simulink model "simple_model"  (R2024a)
settings: Solver=VariableStepAuto  StartTime=0.0  StopTime=150  RelTol=1e-3
InitFcn:
  | A = 100 ;
settings Model: Creator=pc  LastModifiedBy=pc

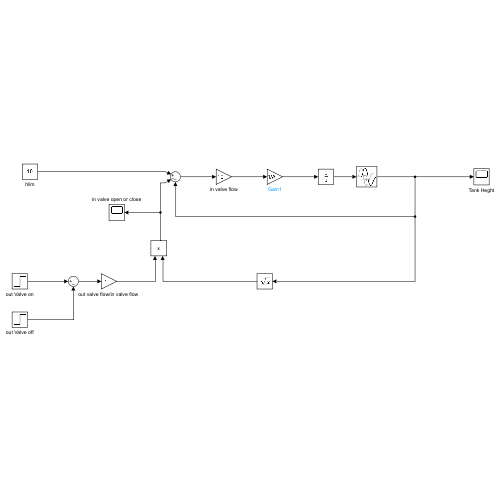
[thumbnail: Simulink's stored preview of the top-level diagram]
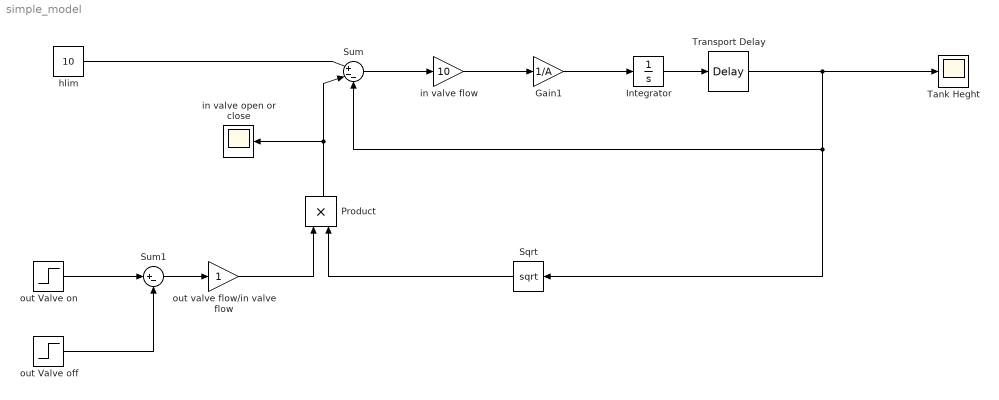
== system simple_model ==
  Gain1 : Gain  Gain=1/A
  Integrator : Integrator  InitialCondition=6
  Product : Product
  Sqrt : Sqrt
  Sum : Sum  Inputs=|+--
  Sum1 : Sum  Inputs=|+-
  Tank Heght : Scope
  Transport Delay : TransportDelay
  hlim : Constant  Value=10
  in valve flow : Gain  Gain=10
  in valve open or close : Scope
  out Valve off : Step  Time=100  SampleTime=0
  out Valve on : Step  Time=40  SampleTime=0
  "out valve flow/in valve flow " : Gain
  wires:
  Integrator/1 -> Transport Delay/1
  Gain1/1 -> Integrator/1
  out Valve on/1 -> Sum1/1
  out Valve off/1 -> Sum1/2
  Sqrt/1 -> Product/2
  Sum1/1 -> "out valve flow/in valve flow "/1
  "out valve flow/in valve flow "/1 -> Product/1
  Product/1 -> in valve open or close/1, Sum/2
  hlim/1 -> Sum/1
  Sum/1 -> in valve flow/1
  in valve flow/1 -> Gain1/1
  Transport Delay/1 -> Tank Heght/1, Sqrt/1, Sum/3
